simulink model "AdaptiveAutocrossDriver"  (R2026b)
settings: Solver=ode4  StopTime=10  FixedStep=0.01
model workspace (MAT data in the model file):
  AADAntiWindupGain = 1
  AADBoundaryGain = 2
  AADBoundaryPreviewDistance = 6
  AADBoundaryReserve = 0.5
  AADBrakePressurePerAcceleration = 10000
  AADCGToFrontAxle = 0.847
  AADCGToRearAxle = 0.693
  AADControlSampleTime = 0.01
  AADCrossTrackGain = 4
  AADCurvatureFilterHalfWindow = 2
  AADCurvatureSafetyFactor = 1
  AADEmergencyBoundaryMargin = 0.25
  AADEnableTC = 1
  AADEnableTV = 1
  AADExitSpeedFeedforwardGain = 0.6
  AADFrontHalfEnvelope = 0.69525
  AADHeadingGain = 1.8
  AADLateralAccelerationLimit = 13.5
  AADMaximumAcceleration = 16
  AADMaximumDeceleration = 8
  AADMaximumSpeed = 32
  AADMaximumSteeringAngle = 0.5
  AADMaximumSteeringPreview = 4
  AADMaximumSteeringRate = 6
  AADMinimumSteeringPreview = 1
  AADMinimumSteeringSpeed = 1
  AADPlanningDeceleration = 6
  AADPreviewBrakeFeedforwardGain = 0.65
  AADPreviewBrakingActivationDistance = 45
  AADPreviewBrakingDecelerationScale = 0.9
  AADPreviewBrakingEnabled = 1
  AADProjectionSearchWindow = 30
  AADRearHalfEnvelope = 0.67525
  AADReferencePathCurvatureBlendEnd = 0.3
  AADReferencePathCurvatureBlendStart = 0.15
  AADReferencePathMaximumBlend = 0
  AADSpeedFeedforwardGain = 0.6
  AADSpeedKi = 0.2
  AADSpeedKp = 4
  AADSpeedPreviewDistance = 190
  AADSpeedPreviewStep = 0.75
  AADSpeedSafetyFactor = 1
  AADSteeringPreviewTime = 0.18
  AADSteeringWheelRatio = 1
  AADWheelbase = 1.54
  PathTrackingAntiWindupGain = 0.5
  PathTrackingBrakePressurePerAcceleration = 10000
  PathTrackingControlSampleTime = 0.01
  PathTrackingCrossTrackGain = 2
  PathTrackingHeadingGain = 1.2
  PathTrackingMaximumAcceleration = 8
  PathTrackingMaximumDeceleration = 8
  PathTrackingMaximumSteeringAngle = 0.5
  PathTrackingMaximumSteeringRate = 4
  PathTrackingMinimumSteeringSpeed = 1
  PathTrackingSpeedKi = 0.25
  PathTrackingSpeedKp = 0.8
  PathTrackingSteeringWheelRatio = 1
  PathTrackingWheelbase = 2
settings Model: DataDictionary=VehicleData.sldd  Creator=Xu Dingyi  LastModifiedBy=29358

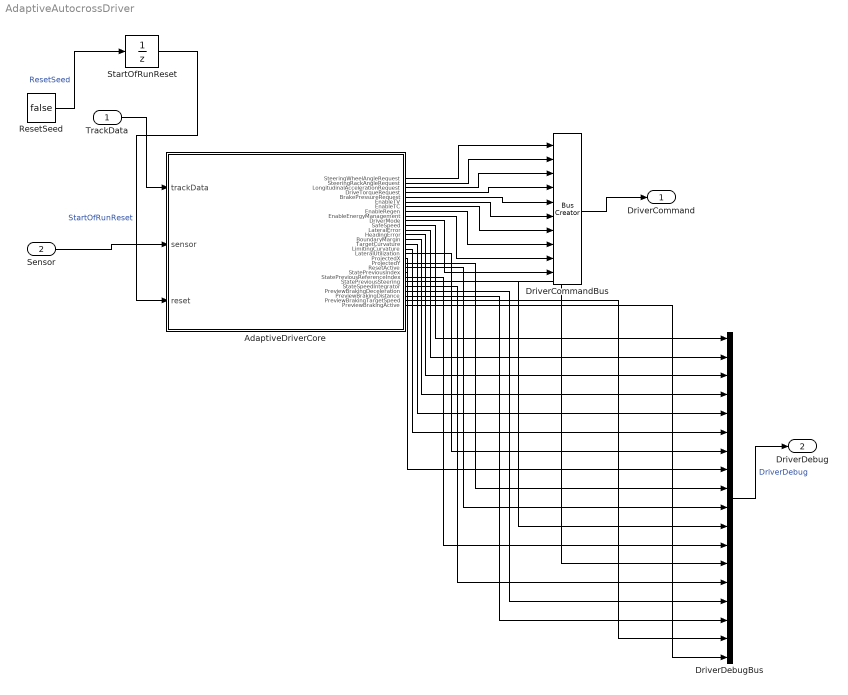
== system AdaptiveAutocrossDriver ==
  TrackData : Inport  OutDataTypeStr=Bus: PathTrackingTrackDataBus
  Sensor : Inport  Port=2  OutDataTypeStr=Bus: SensorBus
  AdaptiveDriverCore : MATLAB Function  TreatAsAtomicUnit=on
  DriverCommandBus : BusCreator  Inputs=10  OutDataTypeStr=Bus: DriverCommandBus
  DriverDebugBus : BusCreator  Inputs=18  OutDataTypeStr=Bus: DriverDebugBus
  ResetSeed : Constant  Value=false  OutDataTypeStr=boolean  SampleTime=AADControlSampleTime
  StartOfRunReset : UnitDelay  InitialCondition=true  SampleTime=AADControlSampleTime
  DriverCommand : Outport  OutDataTypeStr=Bus: DriverCommandBus
  DriverDebug : Outport  Port=2  OutDataTypeStr=Bus: DriverDebugBus
  wires:
  Sensor/1 -> AdaptiveDriverCore/2(sensor)
  AdaptiveDriverCore/1(SteeringWheelAngleRequest) -> DriverCommandBus/1
  AdaptiveDriverCore/2(SteeringRackAngleRequest) -> DriverCommandBus/2
  AdaptiveDriverCore/3(LongitudinalAccelerationRequest) -> DriverCommandBus/3
  AdaptiveDriverCore/4(DriveTorqueRequest) -> DriverCommandBus/4
  AdaptiveDriverCore/5(BrakePressureRequest) -> DriverCommandBus/5
  AdaptiveDriverCore/6(EnableTV) -> DriverCommandBus/6
  AdaptiveDriverCore/7(EnableTC) -> DriverCommandBus/7
  AdaptiveDriverCore/8(EnableRegen) -> DriverCommandBus/8
  AdaptiveDriverCore/9(EnableEnergyManagement) -> DriverCommandBus/9
  AdaptiveDriverCore/10(DriverMode) -> DriverCommandBus/10
  DriverCommandBus/1 -> DriverCommand/1
  TrackData/1 -> AdaptiveDriverCore/1(trackData)
  ResetSeed/1 -> StartOfRunReset/1  "ResetSeed"
  StartOfRunReset/1 -> AdaptiveDriverCore/3(reset)  "StartOfRunReset"
  AdaptiveDriverCore/11(SafeSpeed) -> DriverDebugBus/1
  AdaptiveDriverCore/12(LateralError) -> DriverDebugBus/2
  AdaptiveDriverCore/13(HeadingError) -> DriverDebugBus/3
  AdaptiveDriverCore/14(BoundaryMargin) -> DriverDebugBus/4
  AdaptiveDriverCore/15(TargetCurvature) -> DriverDebugBus/5
  AdaptiveDriverCore/16(LimitingCurvature) -> DriverDebugBus/6
  AdaptiveDriverCore/17(LateralUtilization) -> DriverDebugBus/7
  AdaptiveDriverCore/18(ProjectedX) -> DriverDebugBus/8
  AdaptiveDriverCore/19(ProjectedY) -> DriverDebugBus/9
  AdaptiveDriverCore/20(ResetActive) -> DriverDebugBus/10
  AdaptiveDriverCore/21(StatePreviousIndex) -> DriverDebugBus/11
  AdaptiveDriverCore/22(StatePreviousReferenceIndex) -> DriverDebugBus/12
  AdaptiveDriverCore/23(StatePreviousSteering) -> DriverDebugBus/13
  AdaptiveDriverCore/24(StateSpeedIntegrator) -> DriverDebugBus/14
  DriverDebugBus/1 -> DriverDebug/1  "DriverDebug"
  AdaptiveDriverCore/25(PreviewBrakingDeceleration) -> DriverDebugBus/15
  AdaptiveDriverCore/26(PreviewBrakingDistance) -> DriverDebugBus/16
  AdaptiveDriverCore/27(PreviewBrakingTargetSpeed) -> DriverDebugBus/17
  AdaptiveDriverCore/28(PreviewBrakingActive) -> DriverDebugBus/18

== matlab function AdaptiveAutocrossDriver/AdaptiveDriverCore ==
  settings: updateMethod=DISCRETE  sampleTime=AADControlSampleTime
  data: trackData input; SteeringWheelAngleRequest output; sensor input; SteeringRackAngleRequest output; LongitudinalAccelerationRequest output; DriveTorqueRequest output; BrakePressureRequest output; EnableTV output; EnableTC output; EnableRegen output; EnableEnergyManagement output; DriverMode output; SafeSpeed output; LateralError output; HeadingError output; BoundaryMargin output; TargetCurvature output; LimitingCurvature output; LateralUtilization output; ProjectedX output; ProjectedY output; ResetActive output; StatePreviousIndex output; StatePreviousReferenceIndex output; StatePreviousSteering output; StateSpeedIntegrator output; reset input; PreviewBrakingDeceleration output; PreviewBrakingDistance output; PreviewBrakingTargetSpeed output; PreviewBrakingActive output; AADControlSampleTime parameter; AADWheelbase parameter; AADCGToFrontAxle parameter; AADCGToRearAxle parameter; AADFrontHalfEnvelope parameter; AADRearHalfEnvelope parameter; AADProjectionSearchWindow parameter; AADMinimumSteeringPreview parameter; AADSteeringPreviewTime parameter; AADMaximumSteeringPreview parameter; AADHeadingGain parameter; AADCrossTrackGain parameter; AADBoundaryGain parameter; AADMinimumSteeringSpeed parameter; AADMaximumSteeringAngle parameter; AADMaximumSteeringRate parameter; AADSteeringWheelRatio parameter; AADLateralAccelerationLimit parameter; AADMaximumAcceleration parameter; AADMaximumDeceleration parameter; AADPlanningDeceleration parameter; AADMaximumSpeed parameter; AADSpeedPreviewDistance parameter; AADSpeedPreviewStep parameter; AADCurvatureFilterHalfWindow parameter; AADCurvatureSafetyFactor parameter; AADSpeedSafetyFactor parameter; AADSpeedKp parameter; AADSpeedKi parameter; AADSpeedFeedforwardGain parameter; AADExitSpeedFeedforwardGain parameter; AADPreviewBrakingEnabled parameter; AADPreviewBrakingActivationDistance parameter; AADPreviewBrakeFeedforwardGain parameter; AADPreviewBrakingDecelerationScale parameter; AADAntiWindupGain parameter; AADReferencePathCurvatureBlendStart parameter; AADReferencePathCurvatureBlendEnd parameter; AADReferencePathMaximumBlend parameter; AADBoundaryPreviewDistance parameter; AADBoundaryReserve parameter; AADEmergencyBoundaryMargin parameter; AADEnableTV parameter; AADEnableTC parameter; AADBrakePressurePerAcceleration parameter
function [SteeringWheelAngleRequest, SteeringRackAngleRequest, ...
    LongitudinalAccelerationRequest, DriveTorqueRequest, ...
    BrakePressureRequest, EnableTV, EnableTC, EnableRegen, ...
    EnableEnergyManagement, DriverMode, SafeSpeed, LateralError, ...
    HeadingError, BoundaryMargin, TargetCurvature, ...
    LimitingCurvature, LateralUtilization, ProjectedX, ProjectedY, ...
    ResetActive, StatePreviousIndex, StatePreviousReferenceIndex, ...
    StatePreviousSteering, StateSpeedIntegrator, ...
    PreviewBrakingDeceleration, PreviewBrakingDistance, ...
    PreviewBrakingTargetSpeed, PreviewBrakingActive] = ...
    fcn(trackData, sensor, reset, AADControlSampleTime, AADWheelbase, AADCGToFrontAxle, AADCGToRearAxle, AADFrontHalfEnvelope, AADRearHalfEnvelope, AADProjectionSearchWindow, AADMinimumSteeringPreview, AADSteeringPreviewTime, AADMaximumSteeringPreview, AADHeadingGain, AADCrossTrackGain, AADBoundaryGain, AADMinimumSteeringSpeed, AADMaximumSteeringAngle, AADMaximumSteeringRate, AADSteeringWheelRatio, AADLateralAccelerationLimit, AADMaximumAcceleration, AADMaximumDeceleration, AADPlanningDeceleration, AADMaximumSpeed, AADSpeedPreviewDistance, AADSpeedPreviewStep, AADCurvatureFilterHalfWindow, AADCurvatureSafetyFactor, AADSpeedSafetyFactor, AADSpeedKp, AADSpeedKi, AADSpeedFeedforwardGain, AADExitSpeedFeedforwardGain, AADPreviewBrakingEnabled, AADPreviewBrakingActivationDistance, AADPreviewBrakeFeedforwardGain, AADPreviewBrakingDecelerationScale, AADAntiWindupGain, AADReferencePathCurvatureBlendStart, AADReferencePathCurvatureBlendEnd, AADReferencePathMaximumBlend, AADBoundaryPreviewDistance, AADBoundaryReserve, AADEmergencyBoundaryMargin, AADEnableTV, AADEnableTC, AADBrakePressurePerAcceleration)
%FSAEADAPTIVEAUTOCROSSDRIVERCORE Simulink wrapper for the adaptive driver.
%   This wrapper accepts track geometry and sensor state directly, including
%   the GGV reference-speed ceiling stored in trackData.ReferenceSpeed.

persistent driverState
if isempty(driverState) || logical(reset)
    driverState = initialDriverState();
end

config = struct( ...
    "ControlSampleTime", AADControlSampleTime, ...
    "Wheelbase", AADWheelbase, ...
    "CGToFrontAxle", AADCGToFrontAxle, ...
    "CGToRearAxle", AADCGToRearAxle, ...
    "FrontHalfEnvelope", AADFrontHalfEnvelope, ...
    "RearHalfEnvelope", AADRearHalfEnvelope, ...
    "ProjectionSearchWindow", AADProjectionSearchWindow, ...
    "MinimumSteeringPreview", AADMinimumSteeringPreview, ...
    "SteeringPreviewTime", AADSteeringPreviewTime, ...
    "MaximumSteeringPreview", AADMaximumSteeringPreview, ...
    "HeadingGain", AADHeadingGain, ...
    "CrossTrackGain", AADCrossTrackGain, ...
    "BoundaryGain", AADBoundaryGain, ...
    "MinimumSteeringSpeed", AADMinimumSteeringSpeed, ...
    "MaximumSteeringAngle", AADMaximumSteeringAngle, ...
    "MaximumSteeringRate", AADMaximumSteeringRate, ...
    "SteeringWheelRatio", AADSteeringWheelRatio, ...
    "LateralAccelerationLimit", AADLateralAccelerationLimit, ...
    "MaximumAcceleration", AADMaximumAcceleration, ...
    "MaximumDeceleration", AADMaximumDeceleration, ...
    "PlanningDeceleration", AADPlanningDeceleration, ...
    "MaximumSpeed", AADMaximumSpeed, ...
    "SpeedPreviewDistance", AADSpeedPreviewDistance, ...
    "SpeedPreviewStep", AADSpeedPreviewStep, ...
    "CurvatureFilterHalfWindow", AADCurvatureFilterHalfWindow, ...
    "CurvatureSafetyFactor", AADCurvatureSafetyFactor, ...
    "SpeedSafetyFactor", AADSpeedSafetyFactor, ...
    "SpeedKp", AADSpeedKp, ...
    "SpeedKi", AADSpeedKi, ...
    "SpeedFeedforwardGain", AADSpeedFeedforwardGain, ...
    "ExitSpeedFeedforwardGain", AADExitSpeedFeedforwardGain, ...
    "PreviewBrakingEnabled", AADPreviewBrakingEnabled, ...
    "PreviewBrakingActivationDistance", ...
        AADPreviewBrakingActivationDistance, ...
    "PreviewBrakeFeedforwardGain", AADPreviewBrakeFeedforwardGain, ...
    "PreviewBrakingDecelerationScale", ...
        AADPreviewBrakingDecelerationScale, ...
    "AntiWindupGain", AADAntiWindupGain, ...
    "ReferencePathCurvatureBlendStart", ...
        AADReferencePathCurvatureBlendStart, ...
    "ReferencePathCurvatureBlendEnd", ...
        AADReferencePathCurvatureBlendEnd, ...
    "ReferencePathMaximumBlend", AADReferencePathMaximumBlend, ...
    "BoundaryPreviewDistance", AADBoundaryPreviewDistance, ...
    "BoundaryReserve", AADBoundaryReserve, ...
    "EmergencyBoundaryMargin", AADEmergencyBoundaryMargin, ...
    "EnableTV", AADEnableTV, ...
    "EnableTC", AADEnableTC, ...
    "BrakePressurePerAcceleration", AADBrakePressurePerAcceleration);

[command, driverState, debug] = fsaeAdaptiveAutocrossDriverStep( ...
    trackData, sensor, driverState, config);

SteeringWheelAngleRequest = command.SteeringWheelAngleRequest;
SteeringRackAngleRequest = command.SteeringRackAngleRequest;
LongitudinalAccelerationRequest = ...
    command.LongitudinalAccelerationRequest;
DriveTorqueRequest = command.DriveTorqueRequest;
BrakePressureRequest = command.BrakePressureRequest;
EnableTV = command.EnableTV;
EnableTC = command.EnableTC;
EnableRegen = command.EnableRegen;
EnableEnergyManagement = command.EnableEnergyManagement;
DriverMode = command.DriverMode;
SafeSpeed = debug.SafeSpeed;
LateralError = debug.LateralError;
HeadingError = debug.HeadingError;
BoundaryMargin = debug.BoundaryMargin;
TargetCurvature = debug.TargetCurvature;
LimitingCurvature = debug.LimitingCurvature;
LateralUtilization = debug.LateralUtilization;
ProjectedX = debug.ProjectedX;
ProjectedY = debug.ProjectedY;
ResetActive = logical(reset);
StatePreviousIndex = driverState.PreviousIndex;
StatePreviousReferenceIndex = driverState.PreviousReferenceIndex;
StatePreviousSteering = driverState.PreviousSteering;
StateSpeedIntegrator = driverState.SpeedIntegrator;
PreviewBrakingDeceleration = debug.PreviewBrakingDeceleration;
PreviewBrakingDistance = debug.PreviewBrakingDistance;
PreviewBrakingTargetSpeed = debug.PreviewBrakingTargetSpeed;
PreviewBrakingActive = debug.PreviewBrakingActive;
end

function state = initialDriverState()
state = struct( ...
    "PreviousIndex", 1.0, ...
    "PreviousReferenceIndex", 1.0, ...
    "PreviousSteering", 0.0, ...
    "SpeedIntegrator", 0.0);
end
